simulink model "sxem4"  (R2015b)
settings: Solver=VariableStepAuto  StartTime=0.0  StopTime=1  RelTol=1e-3
settings Model: Creator=hohotulca  LastModifiedBy=hohotulca

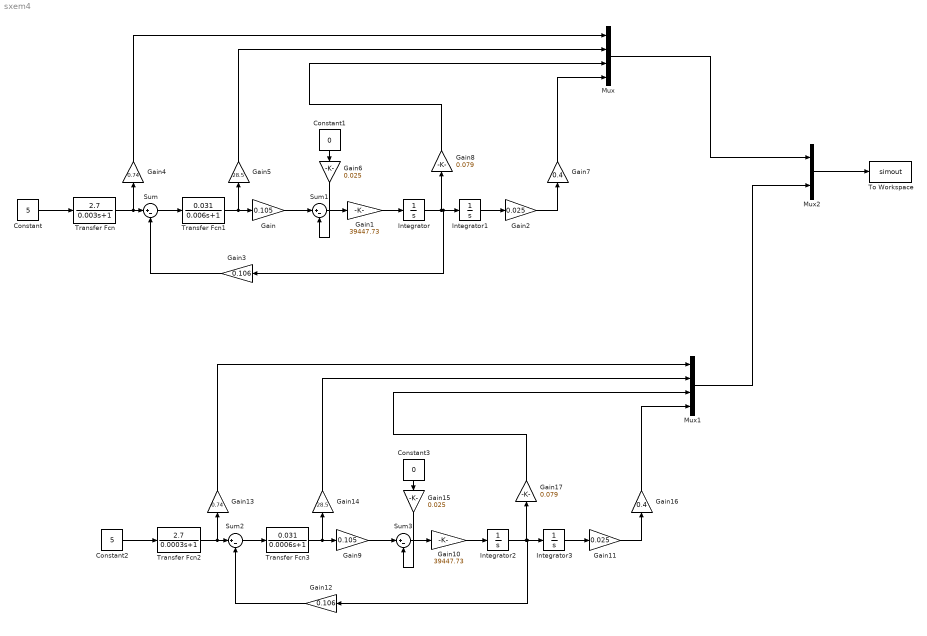
== system sxem4 ==
  Constant : Constant  Value=5
  Constant1 : Constant  Value=0
  Constant2 : Constant  Value=5
  Constant3 : Constant  Value=0
  Gain : Gain  Gain=0.105
  Gain1 : Gain  Gain=39447.73
  Gain10 : Gain  Gain=39447.73
  Gain{2,6,11,15} (4 alike) : Gain  Gain=0.025
  Gain12 : Gain  Gain=0.106
  Gain13 : Gain  Gain=0.74
  Gain14 : Gain  Gain=28.5
  Gain16 : Gain  Gain=0.4
  Gain17 : Gain  Gain=0.079
  Gain3 : Gain  Gain=0.106
  Gain4 : Gain  Gain=0.74
  Gain5 : Gain  Gain=28.5
  Gain7 : Gain  Gain=0.4
  Gain8 : Gain  Gain=0.079
  Gain9 : Gain  Gain=0.105
  Integrator{,1..3} (4 alike) : Integrator
  Mux : Mux
  Mux1 : Mux
  Mux2 : Mux  Inputs=2
  Sum{,1..3} (4 alike) : Sum  Inputs=|+-
  To Workspace : ToWorkspace  VariableName=simout  SaveFormat=Timeseries  SampleTime=-1
  Transfer Fcn : TransferFcn  Numerator=[2.7]  Denominator=[0.003 1]
  Transfer Fcn1 : TransferFcn  Numerator=[0.031]  Denominator=[0.006 1]
  Transfer Fcn2 : TransferFcn  Numerator=[2.7]  Denominator=[0.0003 1]
  Transfer Fcn3 : TransferFcn  Numerator=[0.031]  Denominator=[0.0006 1]
  wires:
  Constant/1 -> Transfer Fcn/1
  Transfer Fcn/1 -> Gain4/1, Sum/1
  Sum/1 -> Transfer Fcn1/1
  Transfer Fcn1/1 -> Gain5/1, Gain/1
  Gain/1 -> Sum1/1
  Sum1/1 -> Gain1/1
  Gain1/1 -> Integrator/1
  Integrator/1 -> Gain3/1, Integrator1/1, Gain8/1
  Integrator1/1 -> Gain2/1
  Gain3/1 -> Sum/2
  Gain6/1 -> Sum1/2
  Constant1/1 -> Gain6/1
  Gain2/1 -> Gain7/1
  Gain4/1 -> Mux/1
  Gain5/1 -> Mux/2
  Gain8/1 -> Mux/3
  Gain7/1 -> Mux/4
  Constant2/1 -> Transfer Fcn2/1
  Transfer Fcn2/1 -> Gain13/1, Sum2/1
  Sum2/1 -> Transfer Fcn3/1
  Transfer Fcn3/1 -> Gain14/1, Gain9/1
  Gain9/1 -> Sum3/1
  Sum3/1 -> Gain10/1
  Gain10/1 -> Integrator2/1
  Integrator2/1 -> Gain12/1, Integrator3/1, Gain17/1
  Integrator3/1 -> Gain11/1
  Gain12/1 -> Sum2/2
  Gain15/1 -> Sum3/2
  Constant3/1 -> Gain15/1
  Gain11/1 -> Gain16/1
  Gain13/1 -> Mux1/1
  Gain14/1 -> Mux1/2
  Gain17/1 -> Mux1/3
  Gain16/1 -> Mux1/4
  Mux/1 -> Mux2/1
  Mux1/1 -> Mux2/2
  Mux2/1 -> To Workspace/1
